simulink model "Q8"  (R2017b)
settings: Solver=VariableStepAuto  StartTime=0.0  StopTime=20  RelTol=1e-3
settings Model: Creator=asus  LastModifiedBy=Kasra

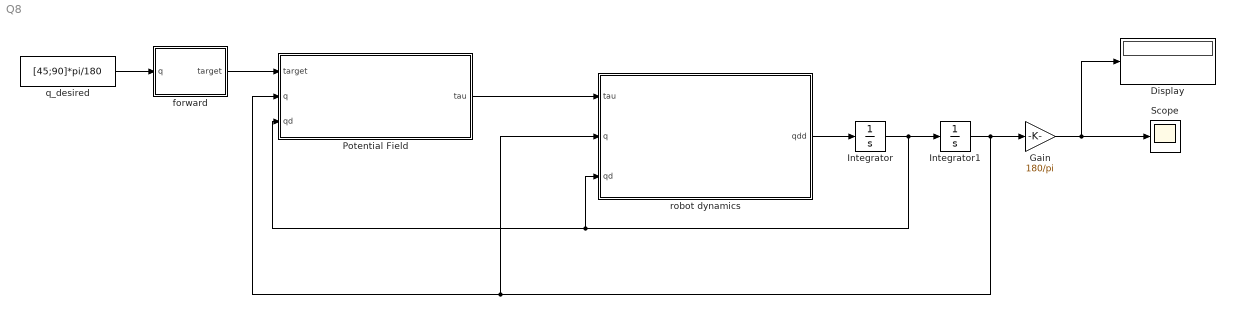
== system Q8 ==
  Display : Display
  Gain : Gain  Gain=180/pi
  Integrator : Integrator  InitialCondition=[0;0]
  Integrator1 : Integrator  InitialCondition=[0;0]*pi/180
  "Potential Field " : MATLAB Function  TreatAsAtomicUnit=on
  Scope : Scope
  "forward " : MATLAB Function  TreatAsAtomicUnit=on
  q_desired : Constant  Value=[45;90]*pi/180
  robot dynamics : MATLAB Function  TreatAsAtomicUnit=on
  wires:
  q_desired/1 -> "forward "/1(q)
  "forward "/1(target) -> "Potential Field "/1(target)
  "Potential Field "/1(tau) -> robot dynamics/1(tau)
  robot dynamics/1(qdd) -> Integrator/1
  Integrator/1 -> "Potential Field "/3(qd), robot dynamics/3(qd), Integrator1/1
  Integrator1/1 -> Gain/1, "Potential Field "/2(q), robot dynamics/2(q)
  Gain/1 -> Display/1, Scope/1

== matlab function Q8/Potential Field  ==
  data: target input; tau output; q input; qd input
function tau = fcn(target, q, qd)

target1=target(:,1);
target2=target(:,2);  

l1 = 0.25;
l2 = 0.12;
lc1 = l1/2;
lc2 = l2/2;
q1 = q(1);
q2 = q(2);

obsa = [0.37;0.1;0]; %obstacle a


o1 = [lc1*cos(q1);lc1*sin(q1);0];
o2 = [l1*cos(q1)+lc2*cos(q1+q2);l1*sin(q1)+lc2*sin(q1+q2);0];

Jc1 = [-lc1*sin(q1), 0;lc1*cos(q1), 0;0, 0];
Jc2 = [-l1*sin(q1)-lc2*sin(q1+q2), -lc2*sin(q1+q2);l1*cos(q1)+lc2*cos(q1+q2), lc2*cos(q1+q2);0, 0];

d = 0.5;
zi = 3000;
B = eye(2)*1;

if norm(o1 - target1)<d
    Fatt1 = -zi*(o1 - target1);
else
    Fatt1 = -zi*(o1 - target1)/norm(o1 - target1);
end

if norm(o2 - target2)<d
    Fatt2 = -zi*(o2 - target2);
else
    Fatt2 = -zi*(o2 - target2)/norm(o2 - target2);
end

p1=o1-obsa;
p2=o2-obsa;
d2=0.1;
n=5;
if norm(p1)<d2
    Frepp11=n*(1/norm(p1)-1/d2)*(1/(norm(p1)^2))*(p1/norm(p1));
else
    Frepp11=[0;0;0];
end

if norm(p2)<d2
    Frepp21=n*(1/norm(p2)-1/d2)*(1/(norm(p2)^2))*(p2/norm(p2));
else
    Frepp21=[0;0;0];
end

 

tau = Jc1'*Fatt1 + Jc2'*Fatt2 - B*qd+Jc1'*Frepp11+Jc2'*Frepp21;

== matlab function Q8/forward  ==
  data: q input; target output
function target = fcn(q)
l1 = 0.25;
l2 = 0.12;
lc1 = l1/2;
lc2 = l2/2;
q1 = q(1);
q2 = q(2);
trg1 = [lc1*cos(q1);lc1*sin(q1);0];
trg2 = [l1*cos(q1)+lc2*cos(q1+q2);l1*sin(q1)+lc2*sin(q1+q2);0];
target =[trg1 trg2];

== matlab function Q8/robot dynamics ==
  data: tau input; qdd output; q input; qd input
function qdd = fcn(tau,q,qd)
l1 = 0.25;
l2 = 0.12;
lc1 = l1/2;
lc2 = l2/2;
I1 = 0.1;
I2 = 0.1;
m1 = 0.1;
m2 = 0.1;
g = 9.81;
q1 = q(1);
q2 = q(2);
qd1 = qd(1);
qd2 = qd(2);

m11 = m1*lc1^(2)+m2*(l1^(2)+lc2^(2)+2*l1*lc2^(2)*cos(q2))+I1+I2;
m12 = m2*(lc2^(2)+l1*lc2*cos(q2))+I2;
m21 = m12;
m22 = m2*lc2^(2)+I2;

h = -m2*l1*l2*sin(q2)*g;

g1 = (m1*lc1+m2*l1)*g*cos(q1)+m2*lc2*g*cos(q1+q2);
g2 = m2*lc2*cos(q1+q2);

C = [h*qd2 h*qd2+h*qd1;-h*qd1 0];
M = [m11 m12;m21 m22];
G = [g1;g2];


qdd = pinv(M)*(tau-C*qd-G);
